simulink model "foc_plant"  (R2026a)
settings: Solver=VariableStepAuto  MaxStep=1/20e3
PreLoadFcn:
  | try, p = fileparts(which(bdroot)); addpath(fullfile(p,'..', 'scripts')); addpath(fullfile(p,'..', 'models')); addpath(p); catch, end; init;
InitFcn:
  | try, p = fileparts(which(bdroot)); addpath(fullfile(p,'..', 'scripts')); addpath(fullfile(p,'..', 'models')); addpath(p); catch, end; init;
undefined symbols (not defined in the file): pmsm
libraries: mcbplantlib x1, autolibpmsminterior x1
settings Model: Creator=probst  LastModifiedBy=niklasprobst
settings DebuggingCC: ParameterPrecisionLossMsg=none

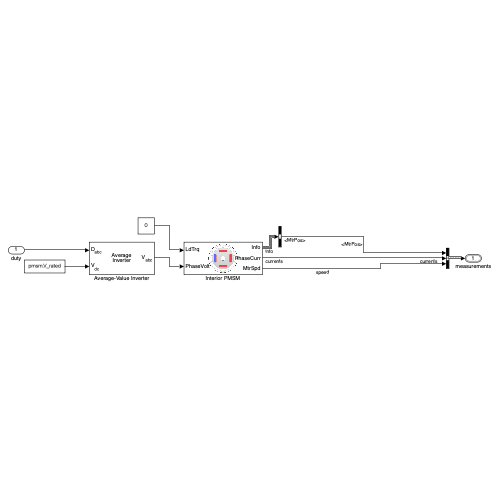
[thumbnail: Simulink's stored preview of the top-level diagram]
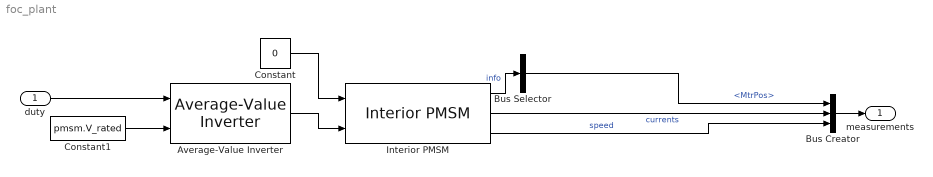
== system foc_plant ==
  duty : Inport
  Average-Value Inverter : mcbplantlib/Average-Value Inverter
      settings: LibrarySourceBlock=mcblib/Electrical Systems/Inverters/Average-Value Inverter
  Bus Creator : BusCreator  Inputs=3  OutDataTypeStr=Bus: measurement  NonVirtualBus=on
  Bus Selector : BusSelector  OutputSignals=MtrPos
  Constant : Constant  Value=0
  Constant1 : Constant  Value=pmsm.V_rated
  Interior PMSM : autolibpmsminterior/Interior PMSM  port_config=Torque  sim_type=Continuous  Ts=0.001  P=pmsm.P  Rs=pmsm.Rs  Ldq=pmsm.Ldq  KConstText=Back-emf constant (Ke):  lambda_pm=0.2205  Ke=pmsm.Ke  mechanical=pmsm.mechanical  idq0=[0 0]  theta_init=0  omega_init=0  KConst=0.2205  lambda_pm_calc=0.2205  Kt=0.07  RefBlkName='autolibpmsminterior/Interior PMSM'  aMode=5
      settings: LibrarySourceBlock=mcblib/Electrical Systems/Motors/Interior PMSM
  measurements : Outport  OutDataTypeStr=Bus: measurement
  wires:
  Constant1/1 -> Average-Value Inverter/2
  Interior PMSM/1 -> Bus Selector/1  "info"
  Average-Value Inverter/1 -> Interior PMSM/2
  Bus Selector/1 -> Bus Creator/1  "<MtrPos>"
  Interior PMSM/2 -> Bus Creator/2  "currents"
  Bus Creator/1 -> measurements/1
  duty/1 -> Average-Value Inverter/1
  Interior PMSM/3 -> Bus Creator/3  "speed"
  Constant/1 -> Interior PMSM/1
